simulink model "generate_test_data_model"  (R2022b)
settings: Solver=FixedStepDiscrete  StartTime=0.0  StopTime=2000  RelTol=1e-3
libraries: aerolibatmos2 x1
settings Model: Creator=86134  LastModifiedBy=86134

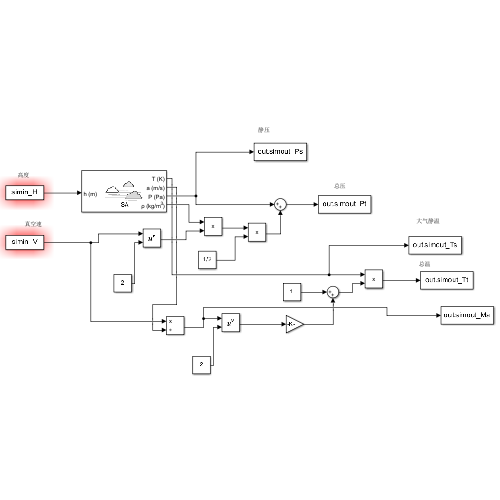
[thumbnail: Simulink's stored preview of the top-level diagram]
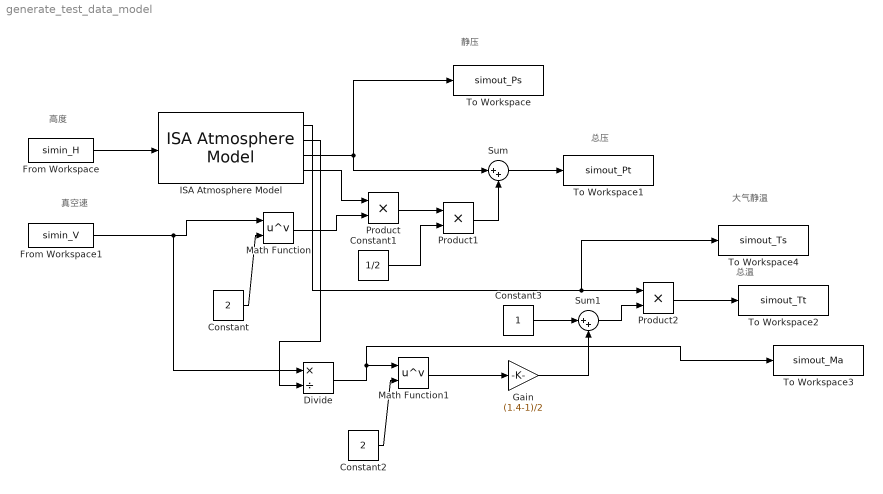
== system generate_test_data_model ==
  note: 大气静温
  note: 总温
  note: 真空速
  note: 高度
  note: 总压
  note: 静压
  Constant : Constant  Value=2
  Constant1 : Constant  Value=1/2
  Constant2 : Constant  Value=2
  Constant3 : Constant
  Divide : Product  Inputs=*/
  From Workspace : FromWorkspace  VariableName=simin_H  SampleTime=0.1
  From Workspace1 : FromWorkspace  VariableName=simin_V  SampleTime=0.1
  Gain : Gain  Gain=(1.4-1)/2
  ISA Atmosphere Model : aerolibatmos2/ISA Atmosphere Model  custom=off  g=9.80665  gamma=1.4  R=287.0531  L=0.0065  h_trop=11000  h_strat=20000  rho0=1.225  P0=101325  T0=288.15  h0=0
  Math Function : Math  Operator=pow
  Math Function1 : Math  Operator=pow
  Product : Product
  Product1 : Product
  Product2 : Product
  Sum : Sum  Inputs=|++
  Sum1 : Sum  Inputs=|++
  To Workspace : ToWorkspace  VariableName=simout_Ps  SaveFormat=Timeseries  SampleTime=0.1
  To Workspace1 : ToWorkspace  VariableName=simout_Pt  SaveFormat=Timeseries  SampleTime=0.1
  To Workspace2 : ToWorkspace  VariableName=simout_Tt  SaveFormat=Timeseries  SampleTime=0.1
  To Workspace3 : ToWorkspace  VariableName=simout_Ma  SaveFormat=Timeseries  SampleTime=-1
  To Workspace4 : ToWorkspace  VariableName=simout_Ts  SaveFormat=Timeseries  SampleTime=-1
  wires:
  From Workspace/1 -> ISA Atmosphere Model/1
  From Workspace1/1 -> Divide/1, Math Function/1
  Constant/1 -> Math Function/2
  ISA Atmosphere Model/4 -> Product/1
  Math Function/1 -> Product/2
  Product/1 -> Product1/1
  Constant1/1 -> Product1/2
  Product1/1 -> Sum/2
  ISA Atmosphere Model/3 -> To Workspace/1, Sum/1
  Sum/1 -> To Workspace1/1
  ISA Atmosphere Model/2 -> Divide/2
  Divide/1 -> To Workspace3/1, Math Function1/1
  Constant2/1 -> Math Function1/2
  Math Function1/1 -> Gain/1
  Gain/1 -> Sum1/2
  Constant3/1 -> Sum1/1
  Sum1/1 -> Product2/2
  ISA Atmosphere Model/1 -> To Workspace4/1, Product2/1
  Product2/1 -> To Workspace2/1
